simulink subsystem "SimpleStateObserver_SubSystem"  (R2021a)
settings: Solver=VariableStepAuto  StartTime=0.0  StopTime=10.0  RelTol=1e-3
undefined symbols (not defined in the file): gbox, Hw, sens, Ts
settings Model: Creator=umberto  LastModifiedBy=utente-A
settings SolverCC: AlgebraicLoopSolver=TrustRegion
settings DebuggingCC: SFMachineParentedDataDiag=warning

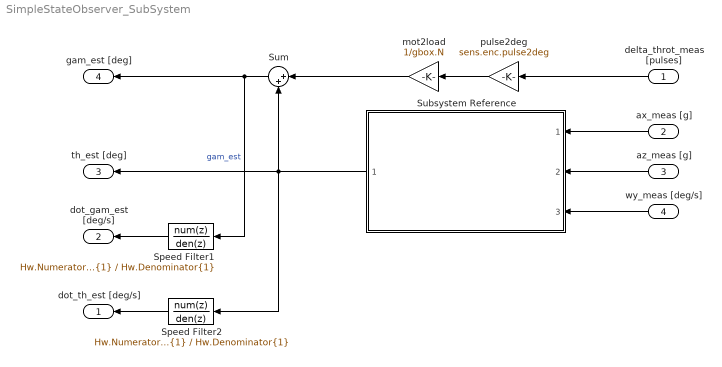
== system SimpleStateObserver_SubSystem ==
  delta_throt_meas [pulses] : Inport
  ax_meas [g] : Inport  Port=2
  az_meas [g] : Inport  Port=3
  wy_meas [deg/s] : Inport  Port=4
  Speed Filter1 : DiscreteTransferFcn  Numerator=Hw.Numerator{1}  Denominator=Hw.Denominator{1}  SampleTime=Ts
  Speed Filter2 : DiscreteTransferFcn  Numerator=Hw.Numerator{1}  Denominator=Hw.Denominator{1}  SampleTime=Ts
  Subsystem Reference : Subsystem  ReferencedSubsystem=CF1_SubSystem
  Sum : Sum  Inputs=|++
  mot2load : Gain  Gain=1/gbox.N
  pulse2deg : Gain  Gain=sens.enc.pulse2deg
  dot_th_est [deg/s] : Outport
  dot_gam_est [deg/s] : Outport  Port=2
  th_est [deg] : Outport  Port=3
  gam_est [deg] : Outport  Port=4
  wires:
  ax_meas [g]/1 -> Subsystem Reference/1
  az_meas [g]/1 -> Subsystem Reference/2
  wy_meas [deg/s]/1 -> Subsystem Reference/3
  delta_throt_meas [pulses]/1 -> pulse2deg/1
  pulse2deg/1 -> mot2load/1
  mot2load/1 -> Sum/1
  Sum/1 -> Speed Filter1/1, gam_est [deg]/1  "gam_est"
  Subsystem Reference/1 -> Sum/2, Speed Filter2/1, th_est [deg]/1
  Speed Filter1/1 -> dot_gam_est [deg/s]/1
  Speed Filter2/1 -> dot_th_est [deg/s]/1
